simulink model "en_linea"  (Simulink 5.0)
settings: Solver=ode45  StartTime=0.0  StopTime=500  RelTol=1e-3
undefined symbols (not defined in the file): ts
libraries: simulink x6, dspstat3 x2
settings Model: LastModifiedBy=pc1  BlockReductionOpt=off  BooleanDataType=off

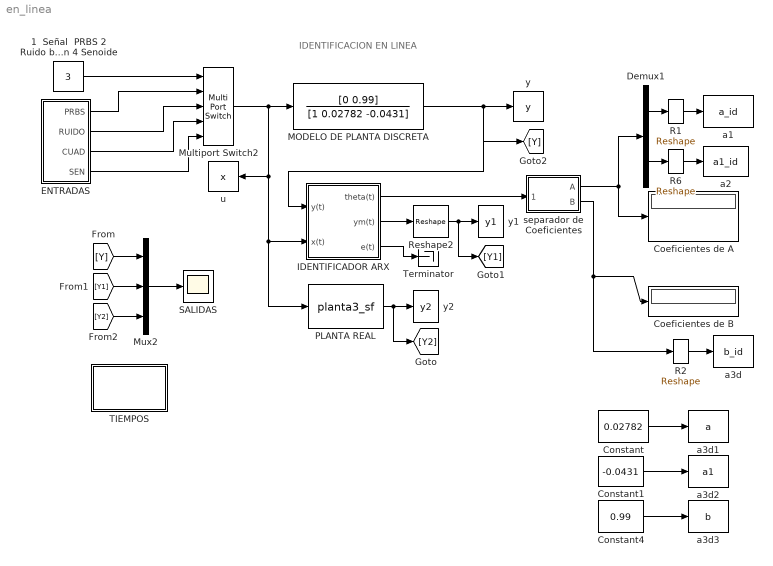
== system en_linea ==
  note: IDENTIFICACION EN LINEA
  1  Señal  PRBS 2 Ruido blanco 3 Escalón 4 Senoide : Constant  Value=3
  Coeficientes de A : Display
  Coeficientes de B : Display
  Constant : Constant  Value=0.02782
  Constant1 : Constant  Value=-0.0431
  Constant4 : Constant  Value=0.99
  Demux1 : Demux  Outputs=2
  ENTRADAS : Subsystem
  IDENTIFICADOR ARX : Subsystem  mask{l=1, ts=ts, nk=1, nb=1, na=2}
      mask prompts: l "valor landa"; ts "valor ts"; nk "valor nk"; nb "valor nb"; na "Valor na"
  MODELO DE PLANTA DISCRETA : DiscreteFilter  Numerator=[0 0.99]  Denominator=[1 0.02782 -0.0431]  SampleTime=ts
  Multiport Switch2 : MultiPortSwitch  SaturateOnIntegerOverflow=on  InputSameDT=on
  Mux2 : Mux  Inputs=3
  PLANTA REAL : S-Function  FunctionName=planta3_sf
  R1 : simulink/Math Operations/Reshape  OutputDimensionality=1-D array  OutputDimensions=[1,1]
  R2 : simulink/Math Operations/Reshape  OutputDimensionality=1-D array  OutputDimensions=[1,1]
  R6 : simulink/Math Operations/Reshape  OutputDimensionality=1-D array  OutputDimensions=[1,1]
  Reshape2 : simulink/Math Operations/Reshape  OutputDimensionality=1-D array  OutputDimensions=[1,1]
  SALIDAS : Scope
  TIEMPOS : Subsystem
  Terminator : Terminator
  a1 : ToWorkspace  VariableName=a_id  SampleTime=ts  SaveFormat=Array
  a2 : ToWorkspace  VariableName=a1_id  SampleTime=ts  SaveFormat=Array
  a3d : ToWorkspace  VariableName=b_id  SampleTime=ts  SaveFormat=Array
  a3d1 : ToWorkspace  VariableName=a  SampleTime=ts  SaveFormat=Array
  a3d2 : ToWorkspace  VariableName=a1  SampleTime=ts  SaveFormat=Array
  a3d3 : ToWorkspace  VariableName=b  SampleTime=ts  SaveFormat=Array
  separador de Coeficientes : Subsystem  mask{na=2, nb=1}
  u : ToWorkspace  VariableName=x  SampleTime=ts  SaveFormat=Array
  y : ToWorkspace  VariableName=y  SampleTime=ts  SaveFormat=Array
  y1 : ToWorkspace  VariableName=y1  SampleTime=ts  SaveFormat=Array
  y2 : ToWorkspace  VariableName=y2  SampleTime=ts  SaveFormat=Array
  wires:
  Multiport Switch2/1 -> u/1, PLANTA REAL/1, IDENTIFICADOR ARX/2(x(t)), MODELO DE PLANTA DISCRETA/1
  MODELO DE PLANTA DISCRETA/1 -> y/1, IDENTIFICADOR ARX/1(y(t)), [Y]
  IDENTIFICADOR ARX/3(e(t)) -> Terminator/1
  separador de Coeficientes/1(A) -> Coeficientes de A/1, Demux1/1
  IDENTIFICADOR ARX/1(theta(t)) -> separador de Coeficientes/1(theta(t))
  separador de Coeficientes/2(B) -> Coeficientes de B/1, R2/1
  PLANTA REAL/1 -> y2/1, [Y2]
  Reshape2/1 -> y1/1, [Y1]
  IDENTIFICADOR ARX/2(ym(t)) -> Reshape2/1
  Mux2/1 -> SALIDAS/1
  1  Señal  PRBS 2 Ruido blanco 3 Escalón 4 Senoide/1 -> Multiport Switch2/1
  ENTRADAS/2(RUIDO) -> Multiport Switch2/3
  ENTRADAS/1(PRBS) -> Multiport Switch2/2
  ENTRADAS/4(SEN) -> Multiport Switch2/5
  Demux1/2 -> R6/1
  R1/1 -> a1/1
  R6/1 -> a2/1
  Demux1/1 -> R1/1
  R2/1 -> a3d/1
  ENTRADAS/3(CUAD) -> Multiport Switch2/4
  [Y] -> Mux2/1
  [Y1] -> Mux2/2
  [Y2] -> Mux2/3
  Constant/1 -> a3d1/1
  Constant1/1 -> a3d2/1
  Constant4/1 -> a3d3/1

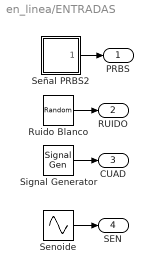
== system en_linea/ENTRADAS ==
  Ruido Blanco : RandomNumber  SampleTime=0
  Senoide : Sin  SampleTime=0
  Señal PRBS2 : Subsystem
  Signal Generator : SignalGenerator  WaveForm=square
  PRBS : Outport
  RUIDO : Outport  Port=2
  CUAD : Outport  Port=3
  SEN : Outport  Port=4
  wires:
  Señal PRBS2/1(u ( t )) -> PRBS/1
  Ruido Blanco/1 -> RUIDO/1
  Signal Generator/1 -> CUAD/1
  Senoide/1 -> SEN/1

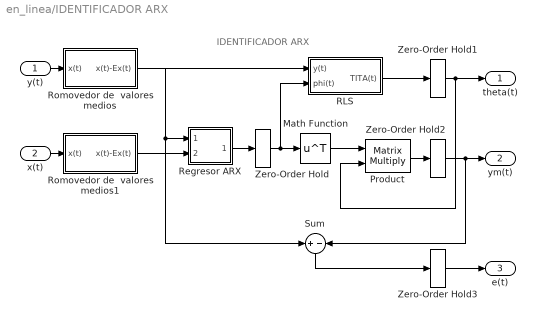
== system en_linea/IDENTIFICADOR ARX ==
  note: IDENTIFICADOR ARX
  y(t) : Inport
  x(t) : Inport  Port=2
  Math Function : Math  Operator=transpose
  Product : Product  Multiplication=Matrix(*)  SaturateOnIntegerOverflow=on  InputSameDT=on
  RLS : Subsystem
  Regresor ARX : Subsystem
  Romovedor de  valores medios : Subsystem
  Romovedor de  valores medios1 : Subsystem
  Sum : Sum  Orientation=down  Inputs=+-  SaturateOnIntegerOverflow=on  InputSameDT=on
  Zero-Order Hold{,1..3} (4 alike) : ZeroOrderHold  SampleTime=ts
  theta(t) : Outport
  ym(t) : Outport  Port=2
  e(t) : Outport  Port=3
  wires:
  Math Function/1 -> Product/1
  Zero-Order Hold3/1 -> e(t)/1
  Product/1 -> Zero-Order Hold2/1
  Zero-Order Hold1/1 -> theta(t)/1, Product/2
  Zero-Order Hold/1 -> RLS/2(phi(t)), Math Function/1
  RLS/1(TITA(t)) -> Zero-Order Hold1/1
  x(t)/1 -> Romovedor de  valores medios1/1(x(t))
  y(t)/1 -> Romovedor de  valores medios/1(x(t))
  Romovedor de  valores medios/1(x(t)-Ex(t)) -> RLS/1(y(t)), Regresor ARX/1(y(t)), Sum/1
  Romovedor de  valores medios1/1(x(t)-Ex(t)) -> Regresor ARX/2(u(t))
  Regresor ARX/1(phi) -> Zero-Order Hold/1
  Zero-Order Hold2/1 -> ym(t)/1, Sum/2
  Sum/1 -> Zero-Order Hold3/1

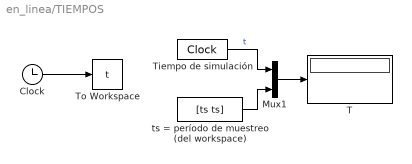
== system en_linea/TIEMPOS ==
  Clock : Clock
      settings: Decimation=10
  Mux1 : Mux  Inputs=2
  T : Display
  Tiempo de simulación : DigitalClock  SampleTime=.1
  To Workspace : ToWorkspace  VariableName=t  SampleTime=ts  SaveFormat=Array
  ts = período de muestreo (del workspace) : FromWorkspace  VariableName=[ts ts]  SampleTime=0
  wires:
  Clock/1 -> To Workspace/1
  ts = período de muestreo (del workspace)/1 -> Mux1/2
  Tiempo de simulación/1 -> Mux1/1  "t"
  Mux1/1 -> T/1

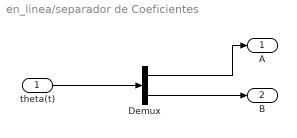
== system en_linea/separador de Coeficientes ==
  theta(t) : Inport
  Demux : Demux  Outputs=[na,nb]
  A : Outport
  B : Outport  Port=2
  wires:
  Demux/1 -> A/1
  theta(t)/1 -> Demux/1
  Demux/2 -> B/1

== system en_linea/ENTRADAS/Señal PRBS2 ==
  Random Number : RandomNumber  SampleTime=0
  Sign : Signum
  Zero-Order Hold : ZeroOrderHold  SampleTime=ts
  u ( t ) : Outport
  wires:
  Zero-Order Hold/1 -> u ( t )/1
  Sign/1 -> Zero-Order Hold/1
  Random Number/1 -> Sign/1

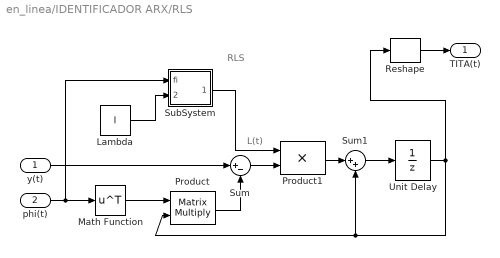
== system en_linea/IDENTIFICADOR ARX/RLS ==
  note: RLS
  note: L(t)
  y(t) : Inport
  phi(t) : Inport  Port=2
  Lambda : Constant  Value=l
  Math Function : Math  Operator=transpose
  Product : Product  Multiplication=Matrix(*)  SaturateOnIntegerOverflow=on  InputSameDT=on
  Product1 : Product  SaturateOnIntegerOverflow=on  InputSameDT=on
  Reshape : simulink/Math Operations/Reshape  OutputDimensionality=Column vector  OutputDimensions=[1,1]
  SubSystem : Subsystem
  Sum : Sum  Inputs=|+-  SaturateOnIntegerOverflow=on  InputSameDT=on
  Sum1 : Sum  Inputs=|++  SaturateOnIntegerOverflow=on  InputSameDT=on
  Unit Delay : UnitDelay  X0=zeros(1,na+nb)'  SampleTime=ts
  TITA(t) : Outport
  wires:
  phi(t)/1 -> SubSystem/1(fi), Math Function/1
  Math Function/1 -> Product/1
  Unit Delay/1 -> Product/2, Sum1/2, Reshape/1
  Product/1 -> Sum/2
  y(t)/1 -> Sum/1
  Sum/1 -> Product1/2
  SubSystem/1(L(t)) -> Product1/1
  Lambda/1 -> SubSystem/2(landa)
  Sum1/1 -> Unit Delay/1
  Product1/1 -> Sum1/1
  Reshape/1 -> TITA(t)/1

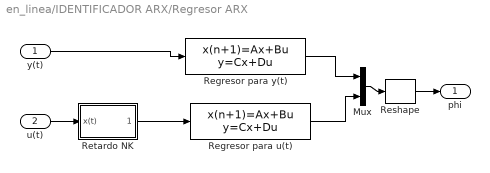
== system en_linea/IDENTIFICADOR ARX/Regresor ARX ==
  y(t) : Inport
  u(t) : Inport  Port=2
  Mux : Mux  Inputs=2
  Regresor para u(t) : DiscreteStateSpace  A=[zeros(1,nb);eye(nb-1,nb)]  B=[1,zeros(1,nb-1)]'  C=eye(nb)  D=[zeros(nb,1)]  SampleTime=ts
  Regresor para y(t) : DiscreteStateSpace  A=[zeros(1,na);eye(na-1,na)]  B=[-1,zeros(1,na-1)]'  C=eye(na)  D=[zeros(na,1)]  SampleTime=ts
  Reshape : simulink/Math Operations/Reshape  OutputDimensionality=Column vector  OutputDimensions=[1,1]
  Retardo NK : Subsystem  mask{nk=nk}
      mask prompts: nk "Valor nk"
  phi : Outport
  wires:
  Reshape/1 -> phi/1
  Retardo NK/1(x(t-nk)) -> Regresor para u(t)/1
  u(t)/1 -> Retardo NK/1(x(t))
  Mux/1 -> Reshape/1
  y(t)/1 -> Regresor para y(t)/1
  Regresor para u(t)/1 -> Mux/2
  Regresor para y(t)/1 -> Mux/1

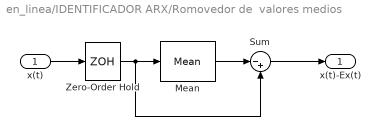
== system en_linea/IDENTIFICADOR ARX/Romovedor de  valores medios ==
  x(t) : Inport
  Mean : dspstat3/Mean  run=on  reset_popup=None
  Sum : Sum  Inputs=|-+  SaturateOnIntegerOverflow=on  InputSameDT=on
  Zero-Order Hold : ZeroOrderHold  SampleTime=ts
  x(t)-Ex(t) : Outport
  wires:
  x(t)/1 -> Zero-Order Hold/1
  Zero-Order Hold/1 -> Mean/1, Sum/2
  Mean/1 -> Sum/1
  Sum/1 -> x(t)-Ex(t)/1

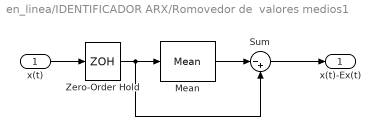
== system en_linea/IDENTIFICADOR ARX/Romovedor de  valores medios1 ==
  x(t) : Inport
  Mean : dspstat3/Mean  run=on  reset_popup=None
  Sum : Sum  Inputs=|-+  SaturateOnIntegerOverflow=on  InputSameDT=on
  Zero-Order Hold : ZeroOrderHold  SampleTime=ts
  x(t)-Ex(t) : Outport
  wires:
  x(t)/1 -> Zero-Order Hold/1
  Zero-Order Hold/1 -> Mean/1, Sum/2
  Mean/1 -> Sum/1
  Sum/1 -> x(t)-Ex(t)/1

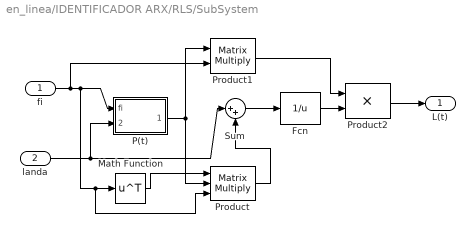
== system en_linea/IDENTIFICADOR ARX/RLS/SubSystem ==
  fi : Inport
  landa : Inport  Port=2
  Fcn : Fcn  Expr=1/u
  Math Function : Math  Operator=transpose
  P(t) : Subsystem
  Product : Product  Inputs=3  Multiplication=Matrix(*)  SaturateOnIntegerOverflow=on  InputSameDT=on
  Product1 : Product  Multiplication=Matrix(*)  SaturateOnIntegerOverflow=on  InputSameDT=on
  Product2 : Product  SaturateOnIntegerOverflow=on  InputSameDT=on
  Sum : Sum  Inputs=|++  SaturateOnIntegerOverflow=on  InputSameDT=on
  L(t) : Outport
  wires:
  Product2/1 -> L(t)/1
  P(t)/1(P(t-1)) -> Product/2, Product1/1
  fi/1 -> P(t)/1(fi), Math Function/1, Product/3, Product1/2
  landa/1 -> P(t)/2(landa), Sum/1
  Math Function/1 -> Product/1
  Product/1 -> Sum/2
  Sum/1 -> Fcn/1
  Fcn/1 -> Product2/2
  Product1/1 -> Product2/1

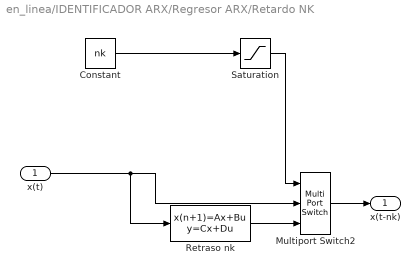
== system en_linea/IDENTIFICADOR ARX/Regresor ARX/Retardo NK ==
  x(t) : Inport
  Constant : Constant  Value=nk
  Multiport Switch2 : MultiPortSwitch  Inputs=2  SaturateOnIntegerOverflow=on  InputSameDT=on
  Retraso nk : DiscreteStateSpace  A=[zeros(1,max(nk,1));eye(max(nk,1)-1,max(nk,1))]  B=[1,zeros(1,max(nk,1)-1)]'  C=[zeros(1,max(nk,1)-1),1]  D=[0]  SampleTime=ts
  Saturation : Saturate  UpperLimit=2  LowerLimit=0
  x(t-nk) : Outport
  wires:
  x(t)/1 -> Retraso nk/1, Multiport Switch2/2
  Multiport Switch2/1 -> x(t-nk)/1
  Retraso nk/1 -> Multiport Switch2/3
  Constant/1 -> Saturation/1
  Saturation/1 -> Multiport Switch2/1

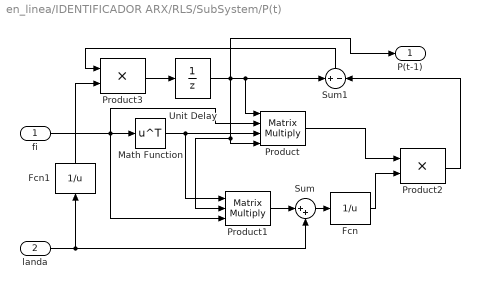
== system en_linea/IDENTIFICADOR ARX/RLS/SubSystem/P(t) ==
  fi : Inport
  landa : Inport  Port=2
  Fcn : Fcn  Expr=1/u
  Fcn1 : Fcn  Orientation=up  Expr=1/u
  Math Function : Math  Operator=transpose
  Product : Product  Inputs=4  Multiplication=Matrix(*)  SaturateOnIntegerOverflow=on  InputSameDT=on
  Product1 : Product  Inputs=3  Multiplication=Matrix(*)  SaturateOnIntegerOverflow=on  InputSameDT=on
  Product2 : Product  SaturateOnIntegerOverflow=on  InputSameDT=on
  Product3 : Product  SaturateOnIntegerOverflow=on  InputSameDT=on
  Sum : Sum  Inputs=|++  SaturateOnIntegerOverflow=on  InputSameDT=on
  Sum1 : Sum  Orientation=up  Inputs=+-  SaturateOnIntegerOverflow=on  InputSameDT=on
  Unit Delay : UnitDelay  X0=100000*eye(na+nb)  SampleTime=ts
  P(t-1) : Outport
  wires:
  Fcn1/1 -> Product3/2
  fi/1 -> Math Function/1, Product/2, Product1/3
  Unit Delay/1 -> P(t-1)/1, Product/4, Product1/2, Product/1, Sum1/1
  Math Function/1 -> Product/3, Product1/1
  Product1/1 -> Sum/1
  landa/1 -> Fcn1/1, Sum/2
  Sum/1 -> Fcn/1
  Fcn/1 -> Product2/2
  Product/1 -> Product2/1
  Sum1/1 -> Product3/1
  Product3/1 -> Unit Delay/1
  Product2/1 -> Sum1/2
